simulink model "sunsensor_valid_logic_test"  (R2016b)
settings: Solver=VariableStepAuto  StartTime=0.0  StopTime=20  RelTol=1e-3
values from neighbouring files (symbols this model uses):
  fsw_params = init_fsw_params()    [sunsensor_processing_test_init.m]    (also in sunsensor_valid_flag_test_init.m)
libraries: simulink x2, sensor_processing_libs x1
settings Model: Creator=Taylor  LastModifiedBy=Taylor

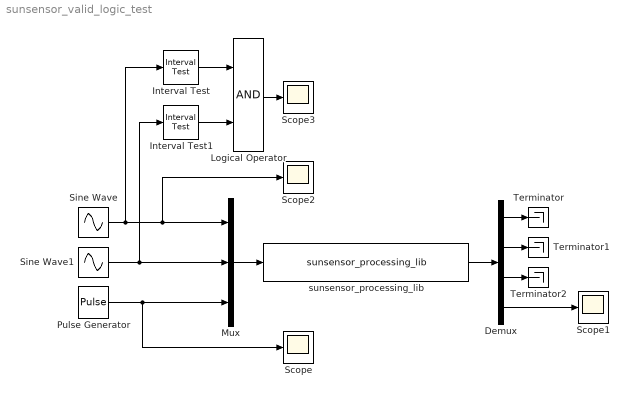
== system sunsensor_valid_logic_test ==
  Demux : Demux
  Interval Test : simulink/Logic and Bit Operations/Interval Test  IntervalClosedRight=on  uplimit=fsw_params.sensor_processing.sunsensor.ang_thresh  IntervalClosedLeft=on  lowlimit=-fsw_params.sensor_processing.sunsensor.ang_thresh  OutDataTypeStr=boolean
  Interval Test1 : simulink/Logic and Bit Operations/Interval Test  IntervalClosedRight=on  uplimit=fsw_params.sensor_processing.sunsensor.ang_thresh  IntervalClosedLeft=on  lowlimit=-fsw_params.sensor_processing.sunsensor.ang_thresh  OutDataTypeStr=boolean
  Logical Operator : Logic  AllPortsSameDT=off  OutDataTypeStr=boolean
  Mux : Mux  Inputs=3
  Pulse Generator : DiscretePulseGenerator  PulseType=Time based  Period=10  PulseWidth=50
  Scope{,1..3} (4 alike) : Scope
  Sine Wave : Sin  Amplitude=90  Phase=-pi/2  SampleTime=0
  Sine Wave1 : Sin  Amplitude=90  Phase=-pi/2  SampleTime=0
  Terminator : Terminator
  Terminator1 : Terminator
  Terminator2 : Terminator
  sunsensor_processing_lib : sensor_processing_libs/sunsensor_processing_lib
  wires:
  Sine Wave/1 -> Interval Test/1, Scope2/1, Mux/1
  Pulse Generator/1 -> Mux/3, Scope/1
  Sine Wave1/1 -> Interval Test1/1, Mux/2
  Demux/4 -> Scope1/1
  Interval Test/1 -> Logical Operator/1
  Interval Test1/1 -> Logical Operator/2
  Logical Operator/1 -> Scope3/1
  Mux/1 -> sunsensor_processing_lib/1
  sunsensor_processing_lib/1 -> Demux/1
  Demux/1 -> Terminator/1
  Demux/2 -> Terminator1/1
  Demux/3 -> Terminator2/1
